simulink model "Lab01es1"  (R2021b)
settings: Solver=VariableStepAuto  StartTime=0.0  StopTime=10.0  RelTol=1e-3
undefined symbols (not defined in the file): c, k, m
libraries: simulink x1
settings Model: Creator=francescafornasier  LastModifiedBy=francescafornasier

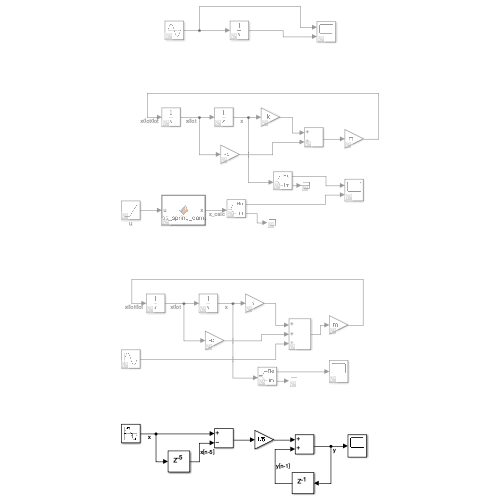
[thumbnail: Simulink's stored preview of the top-level diagram]
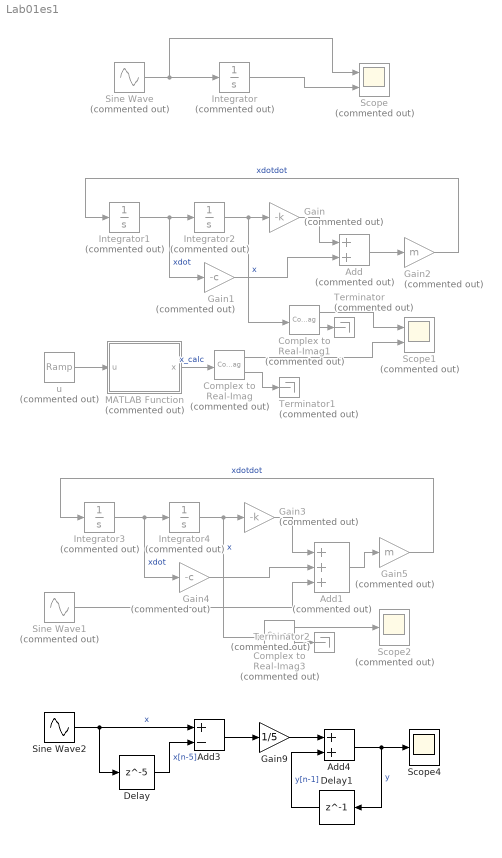
== system Lab01es1 ==
  Add : Sum  Commented=on
  Add1 : Sum  Commented=on  Inputs=+++
  Add3 : Sum  Inputs=+-
  Add4 : Sum
  Complex to Real-Imag : ComplexToRealImag  Commented=on
  Complex to Real-Imag1 : ComplexToRealImag  Commented=on
  Complex to Real-Imag3 : ComplexToRealImag  Commented=on
  Delay : Delay  DelayLength=5  InitialCondition=0
  Delay1 : Delay  DelayLength=1  InitialCondition=0
  Gain : Gain  Commented=on  Gain=-k
  Gain1 : Gain  Commented=on  Gain=-c
  Gain2 : Gain  Commented=on  Gain=m
  Gain3 : Gain  Commented=on  Gain=-k
  Gain4 : Gain  Commented=on  Gain=-c
  Gain5 : Gain  Commented=on  Gain=m
  Gain9 : Gain  Gain=1/5
  Integrator : Integrator  Commented=on
  Integrator1 : Integrator  Commented=on
  Integrator2 : Integrator  Commented=on  InitialCondition=1
  Integrator3 : Integrator  Commented=on
  Integrator4 : Integrator  Commented=on  InitialCondition=1
  MATLAB Function : MATLAB Function  Commented=on  TreatAsAtomicUnit=on
  Scope : Scope  Commented=on  NumInputPorts=2
  Scope1 : Scope  Commented=on  NumInputPorts=2
  Scope2 : Scope  Commented=on
  Scope4 : Scope
  Sine Wave : Sin  Commented=on  SampleTime=0
  Sine Wave1 : Sin  Commented=on  Frequency=2*pi  SampleTime=0
  Sine Wave2 : Sin  Frequency=2*pi  Samples=2*pi/0.1  SampleTime=0.1
  Terminator : Terminator  Commented=on
  Terminator1 : Terminator  Commented=on
  Terminator2 : Terminator  Commented=on
  u : simulink/Sources/Ramp  Commented=on  slope=1  start=0  InitialOutput=0
  wires:
  Sine Wave/1 -> Scope/1, Integrator/1
  Integrator/1 -> Scope/2
  Integrator1/1 -> Gain1/1, Integrator2/1  "xdot"
  Gain2/1 -> Integrator1/1  "xdotdot"
  Integrator2/1 -> Complex to Real-Imag1/1, Gain/1  "x"
  Gain/1 -> Add/1
  Gain1/1 -> Add/2
  Add/1 -> Gain2/1
  u/1 -> MATLAB Function/1(u)
  MATLAB Function/1(x) -> Complex to Real-Imag/1  "x_calc"
  Complex to Real-Imag/2 -> Terminator1/1
  Complex to Real-Imag1/1 -> Scope1/1
  Complex to Real-Imag1/2 -> Terminator/1
  Complex to Real-Imag/1 -> Scope1/2
  Integrator4/1 -> Complex to Real-Imag3/1, Gain3/1  "x"
  Gain3/1 -> Add1/1
  Integrator3/1 -> Gain4/1, Integrator4/1  "xdot"
  Add1/1 -> Gain5/1
  Gain5/1 -> Integrator3/1  "xdotdot"
  Complex to Real-Imag3/2 -> Terminator2/1
  Gain4/1 -> Add1/2
  Sine Wave1/1 -> Add1/3
  Complex to Real-Imag3/1 -> Scope2/1
  Sine Wave2/1 -> Add3/1, Delay/1  "x"
  Delay/1 -> Add3/2  "x[n-5]"
  Add3/1 -> Gain9/1
  Gain9/1 -> Add4/1
  Delay1/1 -> Add4/2  "y[n-1]"
  Add4/1 -> Delay1/1, Scope4/1  "y"

== matlab function Lab01es1/MATLAB Function ==
  data: u input; x output
function x  = mass_spring_damper(u)

k=1;
c=1;
m=1;
wn = sqrt(k/m);
zeta = c/(2*m*wn);
K1 = 1/2-i/(2*sqrt(3));
K2 = 1/2+i/(2*sqrt(3));

y1 = exp(-wn*u*(zeta-sqrt(complex(zeta^2-1))));
y2 = exp(-wn*u*(zeta+sqrt(complex(zeta^2-1))));

x = K1*y1 + K2*y2;
